simulink model "rst_deadzone_facit"  (R2014b)
settings: Solver=ode45  StartTime=0.0  StopTime=20  RelTol=1e-3
undefined symbols (not defined in the file): a1, a2, b1, b2, ea, h, Humusoft, MF624, r1, s0, s1, t0
libraries: rtlib x3
settings Model: Creator=Administrador  LastModifiedBy=kjartan

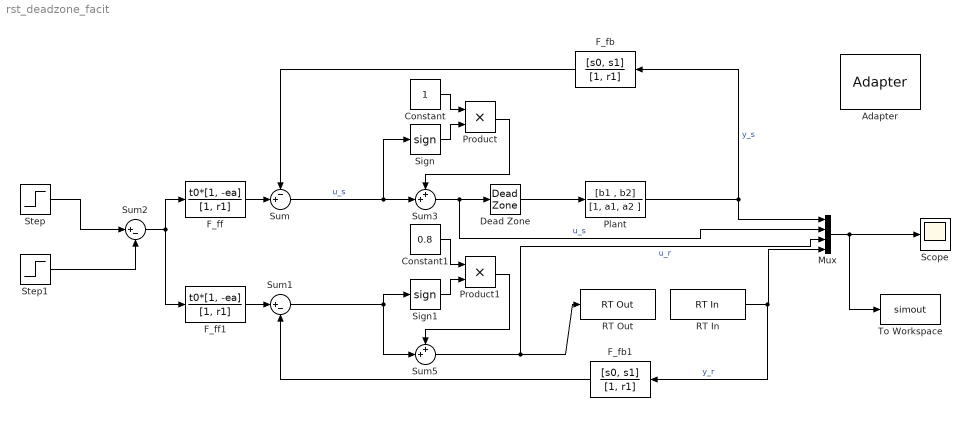
== system rst_deadzone_facit ==
  Adapter : rtlib/Adapter  DriverName=Humusoft/MF624  DriverAddress=4294967295  DriverOptions=0
      settings: AttributesFormatString=Humusoft\nMF624 (auto)
  Constant : Constant
  Constant1 : Constant  Value=0.8
  Dead Zone : DeadZone  LowerValue=-1  UpperValue=1  SaturateOnIntegerOverflow=on
  F_fb : DiscreteTransferFcn  Numerator=[s0, s1]  Denominator=[1, r1]  SampleTime=h
  F_fb1 : DiscreteTransferFcn  Numerator=[s0, s1]  Denominator=[1, r1]  SampleTime=h
  F_ff : DiscreteTransferFcn  Numerator=t0*[1, -ea]  Denominator=[1, r1]  SampleTime=h
  F_ff1 : DiscreteTransferFcn  Numerator=t0*[1, -ea]  Denominator=[1, r1]  SampleTime=h
  Mux : Mux
  Plant : DiscreteTransferFcn  Numerator=[b1 , b2]  Denominator=[1, a1, a2 ]  SampleTime=h
  Product : Product
  Product1 : Product
  RT In : rtlib/RT In  SampleTime=h  Adapter=Adapter  IOClass=Analog Input  Channels=2  SLDataType=double  MaxMissedTicks=100  ShowMissedTicks=off  YieldWhenWaiting=on  AIORange=-10 to 10 V  AIOUnits=Volts  DIOMode=Bit  CIReset=never  CIEdge=rising  CIGate=none  EIQuadrature=quadruple  EIIndexPulse=reset  EIFilterFrequency=Inf  OIOParameters=[]
  RT Out : rtlib/RT Out  SampleTime=h  Adapter=Adapter  IOClass=Analog Output  Channels=2  InitialValue=[0]  FinalValue=[0]  MaxMissedTicks=100  ShowMissedTicks=off  YieldWhenWaiting=on  AIORange=-10 to 10 V  AIOUnits=Volts  DIOMode=Bit  OIOParameters=[]
  Scope : Scope
      settings: ShowLegends=on  TimeRange=20  YMax=15  MaxDataPoints=10000
  Sign : Signum
  Sign1 : Signum
  Step : Step  Time=4  Before=1  After=4  SampleTime=h
  Step1 : Step  Time=10  After=3  SampleTime=h
  Sum : Sum  Inputs=-+|
  Sum1 : Sum  Inputs=|+-
  Sum2 : Sum  Inputs=|+-
  Sum3 : Sum  Inputs=++|
  Sum5 : Sum  Inputs=++|
  To Workspace : ToWorkspace  VariableName=simout  SaveFormat=Timeseries  SampleTime=-1
  wires:
  Mux/1 -> To Workspace/1, Scope/1
  RT In/1 -> Mux/4, F_fb1/1  "y_r"
  Plant/1 -> F_fb/1, Mux/1  "y_s"
  Step1/1 -> Sum2/2
  Step/1 -> Sum2/1
  F_ff/1 -> Sum/2
  F_fb/1 -> Sum/1
  Sum2/1 -> F_ff1/1, F_ff/1
  F_fb1/1 -> Sum1/2
  F_ff1/1 -> Sum1/1
  Sum/1 -> Sign/1, Sum3/2  "u_s"
  Constant/1 -> Product/1
  Sign/1 -> Product/2
  Product/1 -> Sum3/1
  Sum3/1 -> Mux/2, Dead Zone/1  "u_s"
  Sum1/1 -> Sum5/2, Sign1/1
  Constant1/1 -> Product1/1
  Sign1/1 -> Product1/2
  Product1/1 -> Sum5/1
  Sum5/1 -> Mux/3, RT Out/1  "u_r"
  Dead Zone/1 -> Plant/1
